simulink model "week_problem_4"  (R2020b)
settings: Solver=VariableStepAuto  StartTime=0.0  StopTime=10.0  RelTol=1e-3
model workspace (MAT data in the model file):
  B = Simulink.Parameter
  B.Value = 3.5077e-06
  B.DataType = 'auto'
  B.Dimensions = [1 1]
  J = Simulink.Parameter
  J.Value = 3.2284e-06
  J.DataType = 'auto'
  J.Dimensions = [1 1]
  Kd = Simulink.Parameter
  Kd.Value = 0.48976
  Kd.DataType = 'auto'
  Kd.Dimensions = [1 1]
  Ke = Simulink.Parameter
  Ke.Value = 0.0274
  Ke.DataType = 'auto'
  Ke.Dimensions = [1 1]
  Ki = Simulink.Parameter
  Ki.Value = 97.11
  Ki.DataType = 'auto'
  Ki.Dimensions = [1 1]
  Kp = Simulink.Parameter
  Kp.Value = 4810.143
  Kp.DataType = 'auto'
  Kp.Dimensions = [1 1]
  Kt = Simulink.Parameter
  Kt.Value = 0.0274
  Kt.DataType = 'auto'
  Kt.Dimensions = [1 1]
  L = Simulink.Parameter
  L.Value = 2.75e-06
  L.DataType = 'auto'
  L.Dimensions = [1 1]
  N = Simulink.Parameter
  N.Value = 100000
  N.DataType = 'auto'
  N.Dimensions = [1 1]
  R = Simulink.Parameter
  R.Value = 4
  R.DataType = 'auto'
  R.Dimensions = [1 1]
settings Model: Creator=Yeshwanth  LastModifiedBy=Yeshwanth

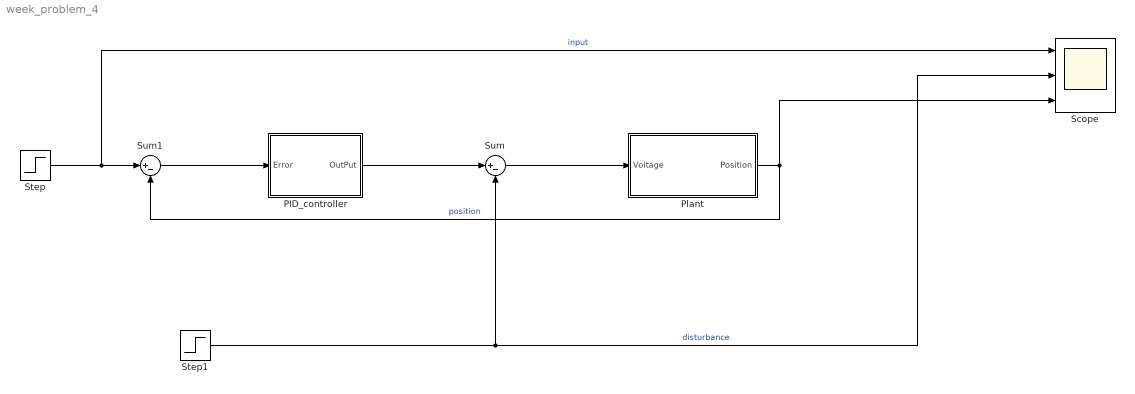
== system week_problem_4 ==
  PID_controller : Subsystem  TreatAsAtomicUnit=on
  Plant : Subsystem
  Scope : Scope  NumInputPorts=3
  Step : Step  Time=0.2  SampleTime=0
  Step1 : Step  Time=0.3  SampleTime=0
  Sum : Sum  Inputs=|+-
  Sum1 : Sum  Inputs=|+-
  wires:
  Sum/1 -> Plant/1(Voltage)
  Plant/1(Position) -> Scope/3, Sum1/2  "position"
  Sum1/1 -> PID_controller/1(Error)
  PID_controller/1(OutPut) -> Sum/1
  Step/1 -> Scope/1, Sum1/1  "input"
  Step1/1 -> Scope/2, Sum/2  "disturbance"

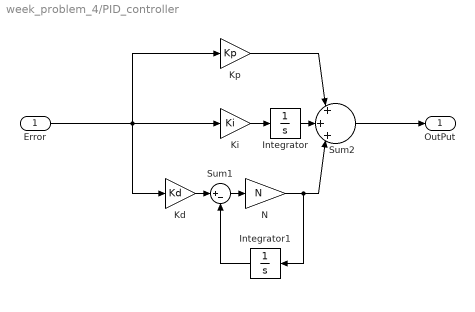
== system week_problem_4/PID_controller ==
  Error : Inport  OutDataTypeStr=double  PortDimensions=1  SampleTime=0
  Integrator : Integrator
  Integrator1 : Integrator
  Kd : Gain  Gain=Kd
  Ki : Gain  Gain=Ki
  Kp : Gain  Gain=Kp
  N : Gain  Gain=N
  Sum1 : Sum  Inputs=|+-
  Sum2 : Sum  Inputs=|+|+|+|
  OutPut : Outport  OutDataTypeStr=double  PortDimensions=1  SampleTime=0
  wires:
  Kd/1 -> Sum1/1
  Error/1 -> Kd/1, Kp/1, Ki/1
  Ki/1 -> Integrator/1
  Kp/1 -> Sum2/1
  Integrator/1 -> Sum2/2
  Sum1/1 -> N/1
  Sum2/1 -> OutPut/1
  N/1 -> Sum2/3, Integrator1/1
  Integrator1/1 -> Sum1/2

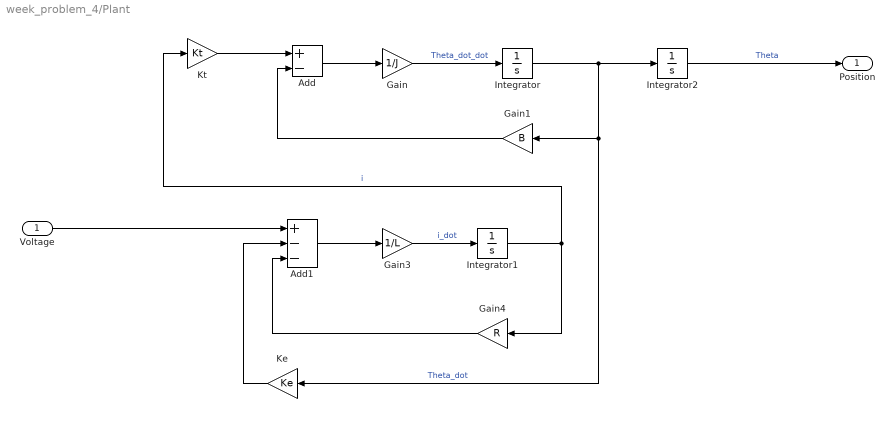
== system week_problem_4/Plant ==
  Voltage : Inport
  Add : Sum  Inputs=+-
  Add1 : Sum  Inputs=+--
  Gain : Gain  Gain=1/J
  Gain1 : Gain  Gain=B
  Gain3 : Gain  Gain=1/L
  Gain4 : Gain  Gain=R
  Integrator : Integrator
  Integrator1 : Integrator
  Integrator2 : Integrator
  Ke : Gain  Gain=Ke
  Kt : Gain  Gain=Kt
  Position : Outport
  wires:
  Voltage/1 -> Add1/1
  Gain1/1 -> Add/2
  Integrator1/1 -> Kt/1, Gain4/1  "i"
  Integrator/1 -> Integrator2/1, Ke/1, Gain1/1  "Theta_dot"
  Kt/1 -> Add/1
  Gain4/1 -> Add1/3
  Add/1 -> Gain/1
  Gain/1 -> Integrator/1  "Theta_dot_dot"
  Ke/1 -> Add1/2
  Add1/1 -> Gain3/1
  Gain3/1 -> Integrator1/1  "i_dot"
  Integrator2/1 -> Position/1  "Theta"
